simulink model "part2_4"  (R2022a)
settings: Solver=VariableStepAuto  StartTime=0.0  StopTime=1.0  RelTol=1e-3
libraries: simulink x2, dspsnks4 x1
settings Model: Creator=marko  LastModifiedBy=marko
settings SolverCC: MaxZcPerStep=1

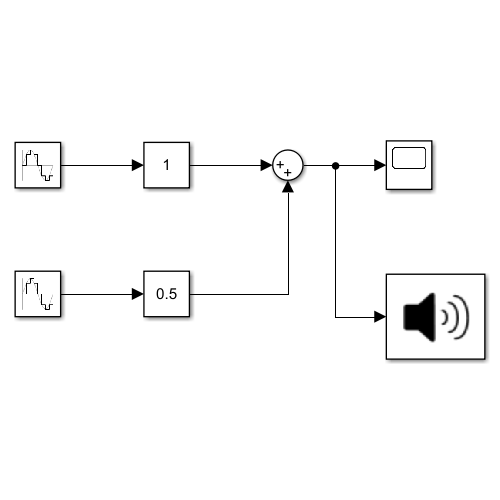
[thumbnail: Simulink's stored preview of the top-level diagram]
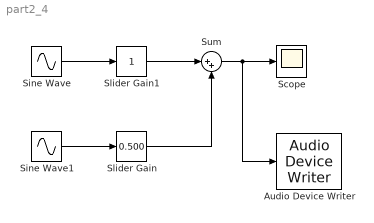
== system part2_4 ==
  Audio Device Writer : dspsnks4/Audio Device Writer  Driver=DirectSound  Device=Speakers (Realtek High Definition Audio(SST))  InheritSampleRate=on  SampleRate=44100  BitDepth=16-bit integer  BufferSize=4096  NumBuffers=10  DefaultOutputChannelMapping=on  OutputChannelMapping=1:2  OutputNumUnderrunSamples=off  DriverIdx=1  DeviceWarnFlag=''
  Scope : Scope
  Sine Wave : Sin  Frequency=2000*pi  Samples=48  SampleTime=1/48000
  Sine Wave1 : Sin  Frequency=4000*pi  Samples=48  SampleTime=1/48000
  Slider Gain : simulink/Math Operations/Slider Gain  gain=0.500  low=0  high=1
  Slider Gain1 : simulink/Math Operations/Slider Gain  gain=1  low=0  high=2
  Sum : Sum  Inputs=|++
  wires:
  Slider Gain1/1 -> Sum/1
  Sine Wave/1 -> Slider Gain1/1
  Sine Wave1/1 -> Slider Gain/1
  Slider Gain/1 -> Sum/2
  Sum/1 -> Audio Device Writer/1, Scope/1
